simulink model "untitled"  (R2023b)
settings: Solver=FixedStepDiscrete  StartTime=0.0  StopTime=10.0  FixedStep=0.01  RelTol=1e-3
settings Model: Creator=MrLove  LastModifiedBy=MrLove

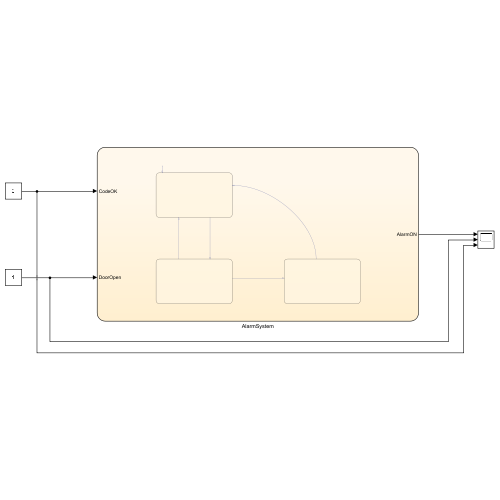
[thumbnail: Simulink's stored preview of the top-level diagram]
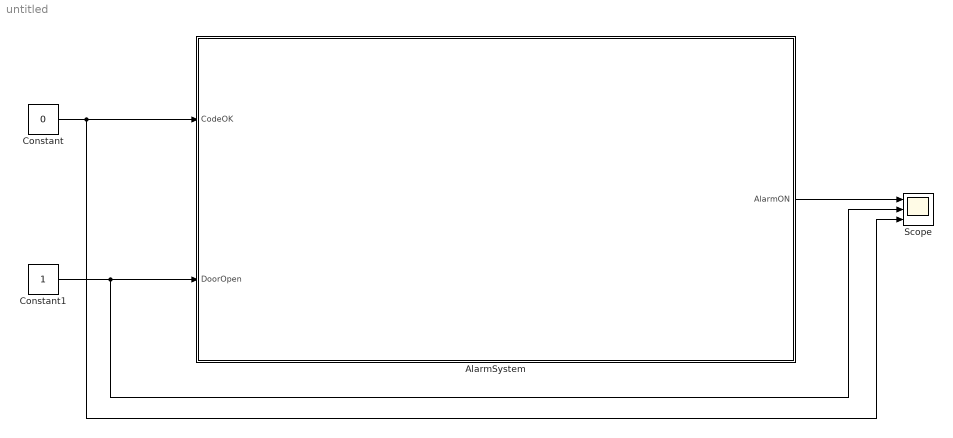
== system untitled ==
  AlarmSystem : Stateflow chart  TreatAsAtomicUnit=on
  Constant : Constant  Value=0
  Constant1 : Constant
  Scope : Scope  NumInputPorts=3
  wires:
  Constant/1 -> AlarmSystem/1(CodeOK), Scope/3
  Constant1/1 -> Scope/2, AlarmSystem/2(DoorOpen)
  AlarmSystem/1(AlarmON) -> Scope/1

== stateflow chart untitled/AlarmSystem ==
  state IDLE
    en:
    AlarmON = false;
  state WAIT
  state ALARM
    en:
    AlarmON = true;
  (default) -> IDLE
  ALARM -> IDLE : [CodeOK == true]
  WAIT -> IDLE [order 1] : [CodeOK == true]
  IDLE -> WAIT : [DoorOpen == true]
  WAIT -> ALARM [order 2] : [after(15,sec)]
  data: CodeOK input; DoorOpen input; AlarmON output
